simulink model "stellaris_lp_irreceive_SONY"  (R2017a)
settings: Solver=ode3  StartTime=0.0  StopTime=0.5  FixedStep=ts  RelTol=1e-3  EnableMultiTasking=on
undefined symbols (not defined in the file or in its folder): ts
libraries: simulink x4, stellaris_lp_lib x4
settings Model: ExtModeTrigDuration=2  Creator=peselnikmg  LastModifiedBy=Nilim
settings DataIOCC: LimitDataPoints=on  SaveFormat=Array  SignalLoggingSaveFormat=ModelDataLogs
settings OptimizationCC: PassReuseOutputArgsAs=Individual arguments  ExpressionDepthLimit=2147483647  MaxStackSize=64
settings DebuggingCC: ParameterTunabilityLossMsg=error  StateNameClashWarn=warning  SFUnexpectedBacktrackingDiag=warning  SFNoUnconditionalDefaultTransitionDiag=warning  SFExecutionAtInitializationDiag=none
settings HardwareCC: ProdBitPerPointer=32  ProdBitPerSizeT=32  ProdBitPerPtrDiffT=32  ProdLargestAtomicInteger=Long  ProdLargestAtomicFloat=Double  ProdWordSize=32  ProdHWDeviceType=ARM Compatible->ARM Cortex
settings ModelReferenceCC: PropagateSignalLabelsOutOfModel=off
settings SFSimCC: MATLABDynamicMemAlloc=off
settings RTWCC: SystemTargetFile=ert.tlc  HardwareBoard=Tiva TM4C123G Launchpad  TLCOptions=-aInlineSetEventsForThisBaseRateFcn=TLC_FALSE -aSuppressMultiTaskScheduler=TLC_FALSE -aRateBasedStepFcn=1  TemplateMakefile=ert_default_tmf  Description=Embedded Coder  GenerateReport=on  RTWVerbose=off  Toolchain=Texas Instruments Code Composer Studio (Tiva)  IncludeHyperlinkInReport=on  LaunchReport=on  GenerateTraceInfo=on  GenerateTraceReport=on  GenerateTraceReportSl=on  GenerateTraceReportSf=on  GenerateTraceReportEml=on
settings CodeAppCC: ForceParamTrailComments=on  IgnoreCustomStorageClasses=off  OperatorAnnotations=on  SimulinkDataObjDesc=on  SFDataObjDesc=on  MATLABFcnDesc=on  CustomSymbolStrType=$N$R$M  InsertBlockDesc=on  MATLABSourceComments=on  InternalIdentifier=Classic
settings ConfigComp: CovMetricSettings=dw  CovHtmlReporting=on  CovSaveCumulativeToWorkspaceVar=on  CovSaveSingleToWorkspaceVar=on  CovExternalEMLEnable=off

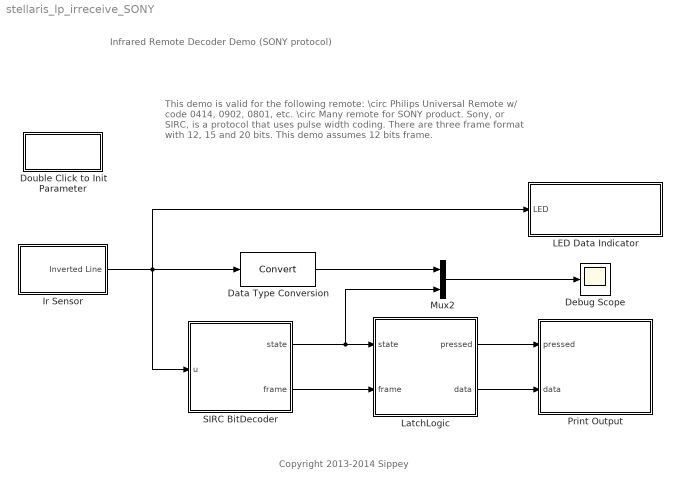
== system stellaris_lp_irreceive_SONY ==
  note: This demo is valid for the following remote:
      | \circ  Philips Universal Remote w/ code 0414, 0902, 0801, etc.
      | \circ  Many remote for SONY product.
      |
      | Sony, or SIRC, is a protocol that uses pulse width coding. There
      | are three frame format with 12, 15 and 20 bits. This demo assumes
      | 12 bits frame.
  note: Infrared Remote Decoder Demo (SONY protocol)
  note: Copyright 2013-2014 Sippey
  Data Type Conversion : DataTypeConversion  SampleTime=ts
  Debug Scope : Scope
  Double Click to Init Parameter : Subsystem
      settings: OpenFcn=ts=0.0001;
      mask Display: fprintf('Double-click');
  Ir Sensor : Subsystem
  LED Data Indicator : Subsystem
  LatchLogic : Stateflow chart  TreatAsAtomicUnit=on
  Mux2 : Mux  Inputs=2
  Print Output : Subsystem
  SIRC BitDecoder : Stateflow chart  TreatAsAtomicUnit=on
  wires:
  Mux2/1 -> Debug Scope/1
  Ir Sensor/1(Inverted Line) -> SIRC BitDecoder/1(u), Data Type Conversion/1, LED Data Indicator/1(LED)
  Data Type Conversion/1 -> Mux2/1
  LatchLogic/1(pressed) -> Print Output/1(pressed)
  LatchLogic/2(data) -> Print Output/2(data)
  SIRC BitDecoder/1(state) -> Mux2/2, LatchLogic/1(state)
  SIRC BitDecoder/2(frame) -> LatchLogic/2(frame)

== system stellaris_lp_irreceive_SONY/Double Click to Init Parameter ==

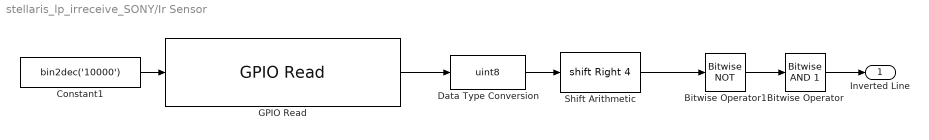
== system stellaris_lp_irreceive_SONY/Ir Sensor ==
  Bitwise Operator : simulink/Logic and Bit Operations/Bitwise Operator  logicop=AND  UseBitMask=on  BitMask=1  BitMaskRealWorld=Stored Integer
  Bitwise Operator1 : simulink/Logic and Bit Operations/Bitwise Operator  logicop=NOT  UseBitMask=off  BitMask=1  BitMaskRealWorld=Stored Integer
  Constant1 : Constant  Value=bin2dec('10000')  OutDataTypeStr=Inherit: Inherit via back propagation
  Data Type Conversion : DataTypeConversion  OutDataTypeStr=uint8  SampleTime=ts
  GPIO Read : stellaris_lp_lib/GPIO/GPIO Read  GPIO_PORTX_BASE=GPIO_PORTF_BASE  SampleTime=-1
      settings: SourceProductName=Run on Stellaris LaunchPad
  Shift Arithmetic : ArithShift  BitShiftNumber=4  BitShiftDirection=Right
  Inverted Line : Outport
  wires:
  Constant1/1 -> GPIO Read/1
  Shift Arithmetic/1 -> Bitwise Operator1/1
  GPIO Read/1 -> Data Type Conversion/1
  Bitwise Operator1/1 -> Bitwise Operator/1
  Bitwise Operator/1 -> Inverted Line/1
  Data Type Conversion/1 -> Shift Arithmetic/1

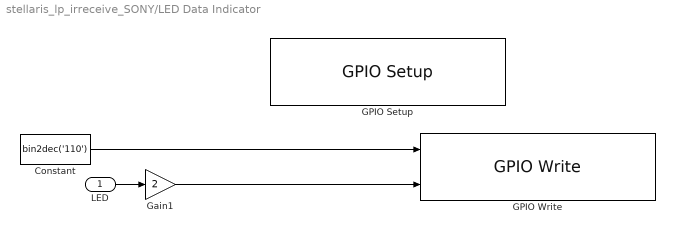
== system stellaris_lp_irreceive_SONY/LED Data Indicator ==
  LED : Inport
  Constant : Constant  Value=bin2dec('110')  OutDataTypeStr=Inherit: Inherit via back propagation
  GPIO Setup : stellaris_lp_lib/GPIO/GPIO Setup  GPIO_PORTX_BASE=GPIO_PORTF_BASE  PinsOutput_0=Input  PinsOutput_1=Output  PinsOutput_2=Output  PinsOutput_3=Output  PinsOutput_4=Input  PinsOutput_5=Input  PinsOutput_6=Input  PinsOutput_7=Input
      settings: SourceProductName=Run on Stellaris LaunchPad
  GPIO Write : stellaris_lp_lib/GPIO/GPIO Write  GPIO_PORTX_BASE=GPIO_PORTF_BASE  SampleTime=-1
      settings: SourceProductName=Run on Stellaris LaunchPad
  Gain1 : Gain  Gain=2  OutDataTypeStr=Inherit: Inherit via back propagation
  wires:
  Constant/1 -> GPIO Write/1
  Gain1/1 -> GPIO Write/2
  LED/1 -> Gain1/1

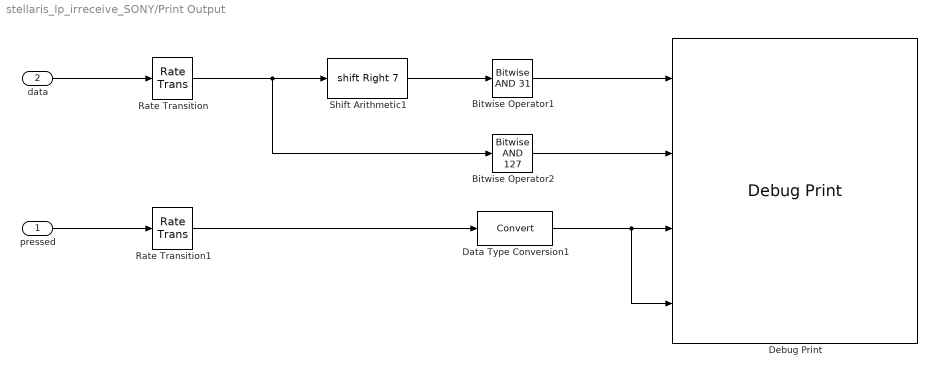
== system stellaris_lp_irreceive_SONY/Print Output ==
  pressed : Inport
  data : Inport  Port=2
  Bitwise Operator1 : simulink/Logic and Bit Operations/Bitwise Operator  logicop=AND  UseBitMask=on  BitMask=31  BitMaskRealWorld=Stored Integer
  Bitwise Operator2 : simulink/Logic and Bit Operations/Bitwise Operator  logicop=AND  UseBitMask=on  BitMask=127  BitMaskRealWorld=Stored Integer
  Data Type Conversion1 : DataTypeConversion
  Debug Print : stellaris_lp_lib/Debug/Debug Print  fmt='addr: %02X, key %d, pressed %d'  sample_time=0.1
      settings: SourceProductName=Run on Stellaris LaunchPad
  Rate Transition : RateTransition
  Rate Transition1 : RateTransition
  Shift Arithmetic1 : ArithShift  BitShiftNumber=7  BitShiftDirection=Right
  wires:
  Rate Transition/1 -> Bitwise Operator2/1, Shift Arithmetic1/1
  Shift Arithmetic1/1 -> Bitwise Operator1/1
  Bitwise Operator1/1 -> Debug Print/1
  Rate Transition1/1 -> Data Type Conversion1/1
  data/1 -> Rate Transition/1
  Data Type Conversion1/1 -> Debug Print/4, Debug Print/3
  pressed/1 -> Rate Transition1/1
  Bitwise Operator2/1 -> Debug Print/2

== stateflow chart stellaris_lp_irreceive_SONY/LatchLogic ==
  state NotPressed
    pressed=0;
    data=0;
  state Pressed
    pressed=1;
  note: If repeat stub is seen, the bit decoder will go
      | to the BitDecoded state once and then timeout.
      | Reset the temporal logic at this time.
  note: timeout after 50ms
      | if a repeat msg have
      | not show up yet
  (default) -> NotPressed
  NotPressed -> Pressed : [state==1]{data=frame;}
  Pressed -> Pressed [order 2] : [state==1]
  Pressed -> NotPressed [order 1] : after(0.05,sec)
  data: state input int32 =0; frame input int32; pressed output int32; data output int32

== stateflow chart stellaris_lp_irreceive_SONY/SIRC BitDecoder ==
  note: bit timeout
  note: Long bit ~ 1.2ms
      | Short bit ~0.6ms
      | Threshold set to 0.9ms
  note: 2.4ms start pulse
      | set 1.8ms as threshold
  note: invalid start bit
  state StartSym
    state = -2;
  state BitWait
    state= -3;
  state Idle
    state = -1;
    frame=0;
  state BitDecoded
    state=-4;
  note: since LSB comes first, every time a bit came
      | the frame buffer shift to right (div 2) and new
      | bit is added to 11th bit ( add 2^11=2048)
  state OutStage
    state=1;
  note: output trigger
      | valid for one tick
  note: 12bit frame is assumed.
  BitWait -> Idle [order 2] : after(5e-3,sec)
  (default) -> Idle
  StartSym -> BitWait [order 1] : after(1.8e-3,sec)
      | [u==0]
      | {nb=0;frame=0;}
  BitWait -> BitDecoded [order 3] : [u==1]{frame=frame/2;nb=nb+1;}
  StartSym -> Idle [order 2] : before(1.8e-3,sec)[u==0]
  BitDecoded -> BitWait [order 2] : before(0.9e-3,sec)[u==0]
  Idle -> StartSym : [u==1]
  BitDecoded -> BitWait [order 1] : after(0.9e-3,sec)[u==0]{frame=frame+2048;}
  OutStage -> Idle
  BitWait -> OutStage [order 1] : [nb>=12]
  data: u input; state output int32 =0; nb local int32; frame output int32
